simulink model "case_1"  (R2018b)
settings: Solver=VariableStepAuto  StartTime=0.0  StopTime=360  RelTol=1e-3
undefined symbols (not defined in the file): a, alpha, gamma1, h0, k
libraries: simulink x15
settings Model: Creator=Romain  LastModifiedBy=Romain

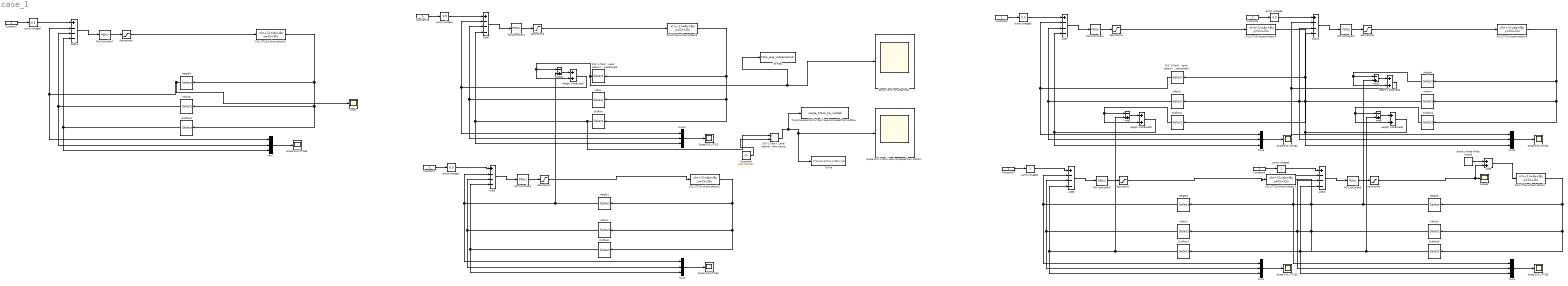
== system case_1 ==
  Add{1,8,12,18} (4 alike) : Sum  Inputs=-+
  Add{3,5..7,10..11,16} (7 alike) : Sum  Inputs=+---
  Add9 : Sum
  Band-Limited White Noise3 : simulink/Sources/Band-Limited White Noise  Cov=[0.00000001]  Ts=0.1  seed=[1]
  Constant{1..5,7,18} (7 alike) : Constant
  Constant6 : Constant  Value=a/(2*sqrt(h0))  SampleTime=-1
  Height 1 attacked{1..4} (4 alike) : Sum
  Height{1,3..6} (5 alike) : Selector  InputPortWidth=3  IndexOptions=Index vector (dialog)  Indices=1  OutputSizes=1
  Inflow{,1..6} (7 alike) : Selector  InputPortWidth=3  IndexOptions=Index vector (dialog)  Indices=2  OutputSizes=1
  Level : Scope
  Mux{1..5,7,10} (7 alike) : Mux  Inputs=3
  Outflow{,1..6} (7 alike) : Selector  InputPortWidth=3  IndexOptions=Index vector (dialog)  Indices=3  OutputSizes=1
  PID Controller{1..7} (7 alike) : simulink/Continuous/PID Controller  Controller=PID  Form=Parallel  TimeDomain=Discrete-time  SampleTime=-1  IntegratorMethod=Forward Euler  FilterMethod=Forward Euler  ControllerParametersSource=internal  P=1  I=1  D=0  UseFilter=off  N=100  TunerSelectOption=Transfer Function Based (PID Tuner App)  InitialConditionSource=internal  InitialConditionForIntegrator=0  InitialConditionForFilter=0  DifferentiatorICPrevScaledInput=0  ExternalReset=none  TrackingMode=off  Kt=1  LimitOutput=off  UpperSaturationLimit=inf  LowerSaturationLimit=-inf  LinearizeAsGain=on  AntiWindupMode=none  Kb=1  POutMin=[]  POutMax=[]  IOutMin=[]  IOutMax=[]  DOutMin=[]  DOutMax=[]  NOutMin=[]  NOutMax=[]  SumOutMin=[]  SumOutMax=[]  SaturationOutMin=[]  SaturationOutMax=[]  PParamMin=[]  PParamMax=[]  IParamMin=[]  IParamMax=[]  DParamMin=[]  DParamMax=[]  NParamMin=[]  NParamMax=[]  KbParamMin=[]  KbParamMax=[]  KtParamMin=[]  KtParamMax=[]  KbOutMin=[]  KbOutMax=[]  KtOutMin=[]  KtOutMax=[]  IntegratorOutMin=[]  IntegratorOutMax=[]  FilterOutMin=[]  FilterOutMax=[]  SumI1OutMin=[]  SumI1OutMax=[]  SumI2OutMin=[]  SumI2OutMax=[]  SumI3OutMin=[]  SumI3OutMax=[]  SumI4OutMin=[]  SumI4OutMax=[]  SumDOutMin=[]  SumDOutMax=[]  DifferentiatorOutMin=[]  DifferentiatorOutMax=[]  FilterDiffOutCoefMin=[]  FilterDiffOutCoefMax=[]  ReciprocalOutMin=[]  ReciprocalOutMax=[]  SumDenOutMin=[]  SumDenOutMax=[]  SumNumOutMin=[]  SumNumOutMax=[]  DivideOutMin=[]  DivideOutMax=[]  IntegratorContinuousStateAttributes=''  IntegratorStateMustResolveToSignalObject=off  IntegratorRTWStateStorageClass=Auto  FilterContinuousStateAttributes=''  FilterStateMustResolveToSignalObject=off  FilterRTWStateStorageClass=Auto  ParallelPVariant=InternalParameters  IdealPVariant=Disabled  IVariant=InternalParameters  DVariant=InternalParameters  IntegratorVariant=Discrete  SatVariant=Disabled  AWVariant=Passthrough  PCopyVariant=Disabled  TRVariant=Disabled  FdbkBlocksVariant=Forward  IdealPFdbkVariant=Disabled  SatFdbkVariant=Disabled  DerivativeFilterVariant=Differentiator  NVariant=Passthrough  NCopyVariant=Disabled_SignalSpec  FilterICVariant=InternalICsDifferentiator  IntegratorICVariant=InternalICs  ExternalResetVariant=Disabled  TRSumVariant=Passthrough  SumFdbkVariant=Disabled  SumVariant=Sum_PID
  "SYS (1-Tank) : Level obtained from outflow sensor" : Product  Inputs=*/
  "SYS (1-Tank) : Level sensor (unattacked)" : Selector  InputPortWidth=3  IndexOptions=Index vector (dialog)  Indices=1  OutputSizes=1
  "SYS (1-Tank) : Level sensor (unattacked)1" : Selector  InputPortWidth=3  IndexOptions=Index vector (dialog)  Indices=1  OutputSizes=1
  SYS LITTLE without attack{1,3..7} (6 alike) : DiscreteStateSpace  A=[-a/(alpha*2*sqrt(h0))]  B=[(gamma1*k)/alpha]  C=[1; 0; a/(2*sqrt(h0))]  D=[0; gamma1*k; 0]  SampleTime=-1
  SYS LITTLE without attack2 : DiscreteStateSpace  A=[-a/(alpha*2*sqrt(h0))]  B=[(0.8*k)/alpha]  C=[1; 0; a/(2*sqrt(h0))]  D=[0; 0.8*k; 0]  SampleTime=-1
  Saturation{1..6,8} (7 alike) : Saturate  UpperLimit=1  LowerLimit=.001
  Scope SYS (1-Tank) level computed from outflow : Scope
  Scope SYS LITTLE{,1..6} (7 alike) : Scope
  Scope3 : Scope
  Sensor level non attacked1 : Scope
  To File : ToFile  Filename=1Tank_level_from_outflow.mat  MatrixName=var_1Tank_level_from_outflow
  To File1 : ToFile  Filename=1Tank_level_unattacked.mat  MatrixName=var_1Tank_level_unattacked
  To Workspace SYS (1-Tank) level computed from outflow : ToWorkspace  VariableName=scope_1Tank_for_matlab  SaveFormat=Timeseries  SampleTime=-1
  pump voltage{1..3,5,7} (5 alike) : simulink/Math Operations/Slider Gain  gain=0.5  low=0  high=1
  pump voltage4 : simulink/Math Operations/Slider Gain  gain=1  low=0  high=1
  pump voltage6 : simulink/Math Operations/Slider Gain  gain=1  low=0  high=1
  wires:
  PID Controller1/1 -> Saturation3/1
  Constant18/1 -> pump voltage1/1
  Mux10/1 -> Scope SYS LITTLE/1
  Add5/1 -> PID Controller1/1
  Inflow/1 -> Add5/3, Mux10/2
  Height 1 attacked2/1 -> Add5/2, Mux10/1
  pump voltage1/1 -> Add5/1
  pump voltage2/1 -> Add3/1
  Add3/1 -> PID Controller2/1
  Constant1/1 -> pump voltage2/1
  PID Controller2/1 -> Saturation1/1
  Saturation1/1 -> SYS LITTLE without attack2/1
  SYS LITTLE without attack2/1 -> Outflow1/1, Inflow1/1, Height1/1
  SYS LITTLE without attack5/1 -> Outflow/1, Inflow/1, "SYS (1-Tank) : Level sensor (unattacked)"/1
  Saturation3/1 -> SYS LITTLE without attack5/1
  Inflow1/1 -> Add3/3, Mux1/2
  Mux1/1 -> Scope SYS LITTLE1/1
  Outflow1/1 -> Add3/4, Mux1/3
  Height1/1 -> Add18/2, Mux1/1, Add3/2
  Add18/1 -> Height 1 attacked2/1
  Saturation4/1 -> SYS LITTLE without attack4/1
  pump voltage4/1 -> Add6/1
  Inflow2/1 -> Add7/3, Mux3/2
  PID Controller4/1 -> Saturation2/1
  Height 1 attacked1/1 -> Add7/4, Mux3/3
  Mux3/1 -> Scope SYS LITTLE2/1
  Saturation2/1 -> SYS LITTLE without attack1/1
  SYS LITTLE without attack4/1 -> Outflow2/1, Inflow2/1, "SYS (1-Tank) : Level sensor (unattacked)1"/1
  SYS LITTLE without attack1/1 -> Outflow3/1, Inflow3/1, Height3/1
  Add7/1 -> PID Controller3/1
  Constant2/1 -> pump voltage4/1
  pump voltage3/1 -> Add7/1
  Inflow3/1 -> Add6/3, Mux2/2
  Mux2/1 -> Scope SYS LITTLE3/1
  PID Controller3/1 -> Saturation4/1
  Constant3/1 -> pump voltage3/1
  Add6/1 -> PID Controller4/1
  Height3/1 -> Mux2/1, Add6/2
  Outflow3/1 -> Add1/2, Add6/4, Mux2/3
  Add1/1 -> Height 1 attacked1/1
  Add8/1 -> Height 1 attacked3/1
  Height 1 attacked3/1 -> Add11/4, Mux5/3
  Saturation6/1 -> SYS LITTLE without attack6/1
  Outflow5/1 -> Add8/2, Add10/4, Mux4/3
  Band-Limited White Noise3/1 -> Add9/1
  SYS LITTLE without attack6/1 -> Outflow4/1, Inflow4/1, Height4/1
  Mux5/1 -> Scope SYS LITTLE4/1
  PID Controller6/1 -> Saturation5/1
  Inflow4/1 -> Add11/3, Mux5/2
  Add9/1 -> SYS LITTLE without attack7/1
  Saturation5/1 -> Add9/2, Scope3/1
  Mux4/1 -> Scope SYS LITTLE5/1
  PID Controller5/1 -> Saturation6/1
  Add10/1 -> PID Controller6/1
  Constant5/1 -> pump voltage5/1
  pump voltage5/1 -> Add11/1
  Inflow5/1 -> Add10/3, Mux4/2
  pump voltage6/1 -> Add10/1
  Add11/1 -> PID Controller5/1
  Constant4/1 -> pump voltage6/1
  SYS LITTLE without attack7/1 -> Outflow5/1, Inflow5/1, Height5/1
  Height 1 attacked4/1 -> Add11/2, Mux5/1
  Height5/1 -> Add12/2, Mux4/1, Add10/2
  Add12/1 -> Height 1 attacked4/1
  Saturation8/1 -> SYS LITTLE without attack3/1
  Inflow6/1 -> Add16/3, Mux7/2
  Outflow6/1 -> Add16/4, Mux7/3
  Mux7/1 -> Scope SYS LITTLE6/1
  SYS LITTLE without attack3/1 -> Outflow6/1, Inflow6/1, Height6/1
  Add16/1 -> PID Controller7/1
  pump voltage7/1 -> Add16/1
  PID Controller7/1 -> Saturation8/1
  Constant7/1 -> pump voltage7/1
  Outflow2/1 -> Height 1 attacked1/2, Add1/1
  Height6/1 -> Level/1, Add16/2, Mux7/1
  "SYS (1-Tank) : Level sensor (unattacked)1"/1 -> Add7/2, Mux3/1
  Outflow4/1 -> Height 1 attacked3/2, Add8/1
  Height4/1 -> Height 1 attacked4/2, Add12/1
  Outflow/1 -> "SYS (1-Tank) : Level obtained from outflow sensor"/1, Add5/4, Mux10/3
  Constant6/1 -> "SYS (1-Tank) : Level obtained from outflow sensor"/2
  "SYS (1-Tank) : Level obtained from outflow sensor"/1 -> To File/1, Scope SYS (1-Tank) level computed from outflow/1, To Workspace SYS (1-Tank) level computed from outflow/1
  "SYS (1-Tank) : Level sensor (unattacked)"/1 -> To File1/1, Sensor level non attacked1/1, Height 1 attacked2/2, Add18/1
